simulink model "Suspension_tractor_example"  (R2017b)
settings: Solver=VariableStepAuto  StartTime=0.0  StopTime=92  RelTol=1e-3
undefined symbols (not defined in the file): dc, ks, m
settings Model: Creator=mm395  LastModifiedBy=mm395

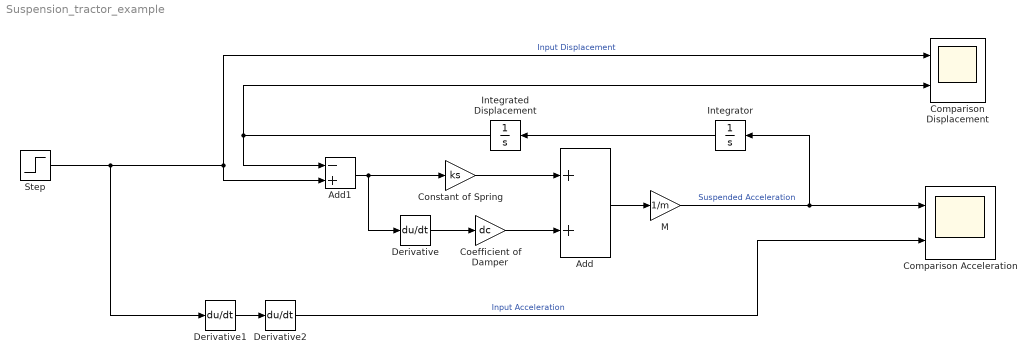
== system Suspension_tractor_example ==
  Add : Sum
  Add1 : Sum  Inputs=-+
  Coefficient of Damper : Gain  Gain=dc
  Comparison Acceleration : Scope  NumInputPorts=2
  Comparison Displacement : Scope  NumInputPorts=2
  Constant of Spring : Gain  Gain=ks
  Derivative : Derivative  CoefficientInTFapproximation=0
  Derivative1 : Derivative  CoefficientInTFapproximation=0
  Derivative2 : Derivative  CoefficientInTFapproximation=0
  Integrated Displacement : Integrator
  Integrator : Integrator
  M : Gain  Gain=1/m
  Step : Step  SampleTime=0
  wires:
  Constant of Spring/1 -> Add/1
  Coefficient of Damper/1 -> Add/2
  Add/1 -> M/1
  Step/1 -> Derivative1/1, Add1/2, Comparison Displacement/1  "Input Displacement"
  M/1 -> Integrator/1, Comparison Acceleration/1  "Suspended Acceleration"
  Add1/1 -> Derivative/1, Constant of Spring/1
  Derivative2/1 -> Comparison Acceleration/2  "Input Acceleration"
  Derivative/1 -> Coefficient of Damper/1
  Integrated Displacement/1 -> Comparison Displacement/2, Add1/1
  Integrator/1 -> Integrated Displacement/1
  Derivative1/1 -> Derivative2/1
